simulink model "stm32f0_can_serial_bridge_binary"  (Simulink 7.3)
settings: Solver=FixedStepDiscrete  SolverMode=SingleTasking  StartTime=0.0  StopTime=10.0  RelTol=1e-3
PreLoadFcn:
  | waijung.modelPreload; % Required for working with Waijung Blockset. Do not remove.
undefined symbols (not defined in the file): LQFP48, STM32F072CB
libraries: simulink x22, stm32f0_can_lib x5, stm32f0_device_config_lib x1
(part 1 of 2)
CloseFcn:
  | waijung.modelClose; % Required for working with Waijung Blockset. Do not remove.
settings Model: Creator=Krisada  LastModifiedBy=Krisada
settings OptimizationCC: OptimizeModelRefInitCode=on  LifeSpan=1
settings HardwareCC: ProdEndianess=LittleEndian  ProdHWDeviceType=ARM Compatible->Cortex - M0  TargetEndianess=LittleEndian  TargetHWDeviceType=ARM Compatible->Cortex - M0
settings RTWCC: SystemTargetFile=stm32f0.tlc  GenerateMakefile=off  TemplateMakefile=ert_default_tmf  Description=STM32F0 Target  ProcessScript=stm32f0_make_rtw_hook
settings CodeAppCC: IgnoreCustomStorageClasses=off
settings STFCustomTargetCC: ModelReferenceCompliant=off  CombineOutputUpdateFcns=on  ERTCustomFileBanners=on  SupportContinuousTime=off  SupportNonInlinedSFcns=off  SystemTargetFile=stm32f0.tlc
settings ERTTargetCC: MultiwordLength=2048  ModelReferenceCompliant=off  ParMdlRefBuildCompliant=off  CompOptLevelCompliant=off  ERTFirstTimeCompliant=off  ModelStepFunctionPrototypeControlCompliant=off  CPPClassGenCompliant=off  ExtModeMexFile=noextcomm  InlinedParameterPlacement=NonHierarchical  ERTSrcFileBannerTemplate=stm32f0_code_template.cgt  ERTHdrFileBannerTemplate=stm32f0_code_template.cgt  ERTDataSrcFileTemplate=stm32f0_code_template.cgt  ERTDataHdrFileTemplate=stm32f0_code_template.cgt  ERTCustomFileTemplate=stm32f0_file_process.tlc

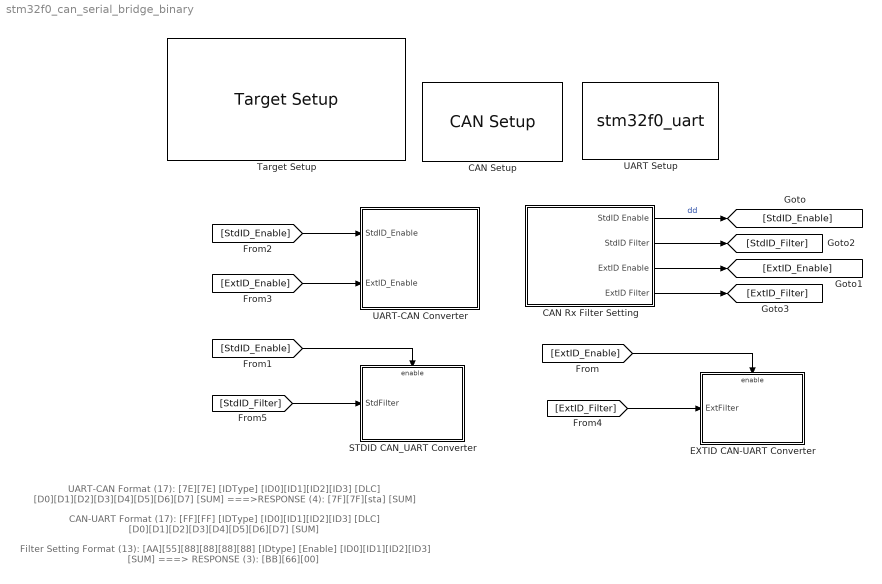
== system stm32f0_can_serial_bridge_binary ==
  note: UART-CAN Format (17): [7E][7E] [IDType] [ID0][ID1][ID2][ID3] [DLC] [D0][D1][D2][D3][D4][D5][D6][D7] [SUM] ===>RESPONSE (4): [7F][7F][sta] [SUM]
  note: CAN-UART Format (17): [FF][FF] [IDType] [ID0][ID1][ID2][ID3] [DLC] [D0][D1][D2][D3][D4][D5][D6][D7] [SUM]
  note: Filter Setting Format (13): [AA][55][88][88][88][88] [IDtype] [Enable] [ID0][ID1][ID2][ID3] [SUM] ===> RESPONSE (3): [BB][66][00]
  CAN Rx Filter Setting : Subsystem
  CAN Setup : stm32f0_can_lib/CAN Setup  conf=Setup  canmodule=1  advance=on  bitrate_select=250000  sjw=1tq  bs1=15tq  bs2=8tq  timingconf=Prescaler  brp=8  bitrate=250000  tq=1.6667e-007  autoretransmission=Enable  remaptxpin=B9  remaprxpin=B8  sampletime=-1  sampletimestr=0.001  blockid=CANSetup  inputarray=[]  inputlabelarray={}  outputarray=[]  outputlabelarray={}  compat=0  confstr="[\"250000\",\"8\",\"B\",\"9\",\"B\",\"8\",\"1tq\",\"15tq\",\"8tq\",\"DISABLE\"]"  presc=8  txportstr=B  txpinstr=9  rxportstr=B  rxpinstr=8  lastmodule=1
  EXTID CAN-UART Converter : Subsystem
  STDID CAN_UART Converter : Subsystem
  Target Setup : stm32f0_device_config_lib/Target Setup  Priority=100  compiler=GNU ARM  previous_compiler=GNU ARM  mcu=STM32F072CB (LQFP48)  mcustr=STM32F072CB  stdlib=STM32F072  clockconfig=STM32F072B-DISCO Default (HSIOSC-8MHz/HCLK-48MHz)  system_stm32f0xx_c_path=F:\trunk\targets\stm32f0_target\stm32f0\utils\STM32F0xx_AN4055\stm32f0_default\hsi8mhz_pll_hclk48mhz  showmemoryconfiguration=off  stacksize=0x400  heapsize=0x200  enableautocompiledownload=on  fullchiperase=off  programmerinterface=aMG USB Connect  editctrlstr=off  compilercontrolstr=$(patsubst %, -I%, .) -mcpu=cortex-m0 -mthumb -mabi=aapcs -Wall -O3 -mfloat-abi=soft -ffunction-sections -fdata-sections -fno-strict-aliasing -fno-builtin --short-enums  assemblercontrolstr=$(patsubst %, -I%, .) -mcpu=cortex-m0 -mtune=cortex-m0 -mthumb -Wall -O3 -Wa,-amhls=$(<:.s=.lst) -D__STACK_SIZE=$(STACK_SIZE) -D__HEAP_SIZE=$(HEAP_SIZE)  linkercontrolstr="-T$(LD_SCRIPT) -Wl,-Map=$(MAP),--cref,--no-warn-mismatch -mcpu=cortex-m0 -mthumb  -Wall -O3 -mabi=aapcs -lc -specs=nosys.specs"  runafterdownload=on  execprofile=None  profileruart=3  profilerbaud=500000  profilertxpin=Not used  profilerinitstr=0.001,48000000,48000,500000,0  manualsetsampletime=on  sampletime=0.001  blockid=TargetSetup  systickreloadvalue=48000  hseval=8000000  lastprofileruart=3  hclk=48000000  flashorigin=0x8000000  flashlength=128k  ramorigin=0x20000000  ramlength=16k  useextram=off
  UART Setup : S-Function  FunctionName=stm32f0_uart  Parameters=conf,inputporttype,inputportwidth,outputporttype,outputportwidth,asciiheader,optionstring,headerstring,terminatorstring,asciidatatypestring,sampletime,blockid  EnableBusSupport=off  mask(stm32f0_uart){conf=Setup, uartmodule=1, baudrate=115200, databits=8, parity=No, stopbit=1, remaptxpin=A9, remaprxpin=A10, flowcontrol=None, remapctspin=Not used, remaprtspin=Not used, advanceoptions=on, rxbuffersize=128, txbuffersize=128, transfer=Non-Blocking, packetmode=Binary, binheader='7E 7E', binterminator='03 03', porttype_double=1, porttype_single=1, porttype_int8=0, porttype_uint8=0, porttype_int16=0, porttype_uint16=1, porttype_int32=0, porttype_uint32=0, asciiformat='%1.2f', rx_asciiterminator=CR (0x0D - "\r"), tx_asciiterminator=CR (0x0D - "\r"), storagename=<empty>, varname=, asciiheader=, sampletime=-1, enablecustomportlabel=off, cinputportlabel=de, coutputportlabel=fff,ff,sdfsd, portpinstr=0, blockid=UARTSetup, inputporttype=[], inputportwidth=[], inputportlabel={}, outputporttype=[], outputportwidth=[], outputportlabel={}, compat=0, optionstring=["1", "1", "A", "9", "1", "A", "10", "0", "*", "*", "0", "*", "*", "1", "1", "", "", "115200", "8", "No", "1", "None", "3", "2", "128", "128", "Binary", "Non-Blocking", ""], headerstring=[], terminatorstring=[], asciidatatypestring=[], lastmodule=1}
      mask prompts: conf "Configuration"; uartmodule "UART Module"; baudrate "Baud rate (bps)"; databits "Data bits"; stopbit "Stop bit"; remaptxpin "Tx pin"; remaprxpin "Rx pin"; flowcontrol "Hardware flow control"; remapctspin "HW Flow control, CTS Pin"; remaprtspin "HW Flow control, RTS Pin"; advanceoptions "Advance options"; rxbuffersize "Rx buffer size (bytes)"; txbuffersize "Tx buffer size (bytes)"; packetmode "Packet mode"; binheader "Binary header (example: '7E 7E')"; binterminator "Binary terminator (example: '03 03')"; porttype_double "Number of data port, type DOUBLE"; porttype_single "Number of data port, type SINGLE"; porttype_int8 "Number of data port, type INT8"; porttype_uint8 "Number of data port, type UINT8"; porttype_int16 "Number of data port, type INT16"; porttype_uint16 "Number of data port, type UINT16"; porttype_int32 "Number of data port, type INT32"; porttype_uint32 "Number of data port, type UINT32"; asciiformat "Ascii format"; rx_asciiterminator "End of packet"; tx_asciiterminator "End of packet"; storagename "Buffer"; varname "Var name"; asciiheader "Ascii header (printf format)"; sampletime "Sample time (sec)"; enablecustomportlabel "Enable custom port labels (Ex. In1, In2, In3)"; cinputportlabel "Custom input port labels (Ex. In1, In2, In3)"; coutputportlabel "Custom output port labels (Ex. Out1, Out2, Out3)"; portpinstr "Port Pin String"; blockid "Block ID"; inputporttype "Input Port Type"; inputportwidth "Input Port Width"; inputportlabel "Input Port Label"; outputporttype "Output Port Type"; outputportwidth "Output Port Width"; outputportlabel "Output port label"; compat "Compatibility (Reserved for future use)"; optionstring "String(s) to be passed to TLC"; lastmodule "Last module selected"
      mask help:
      | Default configuration for aMG USB Connect board:
      |  - UART module: 1
      |  - Tx pin: A9
      |  - Rx pin: A10
      |
      | Advance options
      |  - Rx buffer size (bytes): max packet length can be received via DMA.
      |  - Tx buffer size (bytes): max packet length can be transmit via DMA.
      mask init:
      | stm32f0_uart_callback('init');
      mask Help: web(fullfile(waijungdocroot,'stm32f0_uart_setup.htm'), '-browser')
      mask StyleString: popup(Setup|Tx|Rx),popup(1|2|3|4),edit,popup(8),popup(No|Odd|Even),popup(0.5|1|1.5|2),popup(Not used|A9|B6),popup(Not used|A10|B7),popup(None|RTS|CTS|RTS/CTS),popup(Not used|A11),popup(Not used|A12),checkbox,popup(16|32|64|128|256|512),popup(16|32|64|128|256|512),popup(Blocking|Non-Blocking),popup(Ascii|Binary|String Buffer),edit,edit,edit,edit,edit,edit,edit,edit,edit,edit,edit,popup(CR (0x0D - "\r")|LF (0x0A - "\n")|CRLF (0x0D 0x0A - "\r\n")),popup(CR (0x0D - "\r")|LF (0x0A - "\n")|CRLF (0x0D 0x0A - "\r\n")|None),popup(<empty>),edit,edit,edit,checkbox,edit,edit,edit,edit,edit,edit,edit,edit,edit,edit,edit,edit,edit,edit,edit,edit
      mask CallbackString: stm32f0_uart_callback('conf');|stm32f0_uart_callback('uartmodule');|||||||stm32f0_uart_callback('flowcontrol');|||stm32f0_uart_callback('advanceoptions');|||stm32f0_uart_callback('conf');|stm32f0_uart_callback('conf');|stm32f0_uart_callback('binheader');|stm32f0_uart_callback('binterminator');|||||||||stm32f0_uart_callback('asciiformat');|||stm32f0_uart_callback('storagename');|||stm32f0_uart_callback('sampletime');|stm32f0_uart_callback('enablecustomportlabel');|stm32f0_uart_callback('conf');|stm32f0_uart_callback('conf');||stm32f0_uart_callback('blockid');||||||||||||
      mask Display: text(0.5, 0.5, 'Module: USART1_Setup\nBaud (Bps): 115200\nDMA Buffer: 128/128\nTx/Rx Pin: A9/A10','ver','middle','hor','center');
  UART-CAN Converter : Subsystem
  wires:
  CAN Rx Filter Setting/1(StdID Enable) -> [StdID_Enable]  "dd"
  CAN Rx Filter Setting/3(ExtID Enable) -> [ExtID_Enable]
  CAN Rx Filter Setting/2(StdID Filter) -> [StdID_Filter]
  CAN Rx Filter Setting/4(ExtID Filter) -> [ExtID_Filter]
  [ExtID_Enable] -> EXTID CAN-UART Converter/Enable
  [StdID_Enable] -> STDID CAN_UART Converter/Enable
  [StdID_Enable] -> UART-CAN Converter/1(StdID_Enable)
  [ExtID_Enable] -> UART-CAN Converter/2(ExtID_Enable)
  [ExtID_Filter] -> EXTID CAN-UART Converter/1(ExtFilter)
  [StdID_Filter] -> STDID CAN_UART Converter/1(StdFilter)

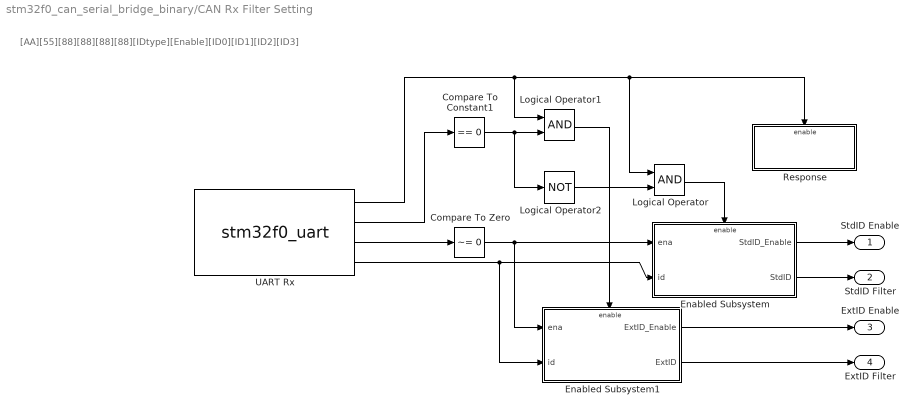
== system stm32f0_can_serial_bridge_binary/CAN Rx Filter Setting ==
  note: [AA][55][88][88][88][88][IDtype][Enable][ID0][ID1][ID2][ID3]
  Compare To Constant1 : simulink/Logic and Bit Operations/Compare To Constant  SystemSampleTime=-1  relop===  const=0  LogicOutDataTypeMode=uint8  ZeroCross=off
  Compare To Zero : simulink/Logic and Bit Operations/Compare To Zero  SystemSampleTime=-1  relop=~=  LogicOutDataTypeMode=uint8  ZeroCross=off
  Enabled Subsystem : Subsystem  TreatAsAtomicUnit=on
  Enabled Subsystem1 : Subsystem  TreatAsAtomicUnit=on
  Logical Operator : Logic  AllPortsSameDT=off  OutDataTypeMode=boolean  LogicDataType=fixdt(0, 8)  OutDataTypeStr=boolean
  Logical Operator1 : Logic  AllPortsSameDT=off  OutDataTypeMode=boolean  LogicDataType=fixdt(0, 8)  OutDataTypeStr=boolean
  Logical Operator2 : Logic  Operator=NOT  AllPortsSameDT=off  OutDataTypeMode=boolean  LogicDataType=fixdt(0, 8)  OutDataTypeStr=boolean
  Response : Subsystem  TreatAsAtomicUnit=on
  UART Rx : S-Function  FunctionName=stm32f0_uart  Parameters=conf,inputporttype,inputportwidth,outputporttype,outputportwidth,asciiheader,optionstring,headerstring,terminatorstring,asciidatatypestring,sampletime,blockid  EnableBusSupport=off  mask(stm32f0_uart){conf=Rx, uartmodule=1, baudrate=115200, databits=8, parity=No, stopbit=1, remaptxpin=A9, remaprxpin=A10, flowcontrol=None, remapctspin=Not used, remaprtspin=Not used, advanceoptions=off, rxbuffersize=64, txbuffersize=64, transfer=Non-Blocking, packetmode=Binary, binheader='AA 55 88 88 88 88', binterminator='', porttype_double=0, porttype_single=0, porttype_int8=0, porttype_uint8=2, porttype_int16=0, porttype_uint16=0, porttype_int32=0, porttype_uint32=1, asciiformat='cantx,extid=%u,dlc=%x,data=%x,%x,%x,%x,%x,%x,%x,%x', rx_asciiterminator=CRLF (0x0D 0x0A - "\r\n"), tx_asciiterminator=LF (0x0A - "\n"), storagename=<empty>, varname=, asciiheader=, sampletime=inf, enablecustomportlabel=on, cinputportlabel=de, coutputportlabel=IDtype,Enable,ID, portpinstr=0, blockid=CANRxFilterSettingUARTRx, inputporttype=[], inputportwidth=[], inputportlabel={}, outputporttype=[3 3 3 7], outputportwidth=[], outputportlabel={'READY' 'IDtype' 'Enable' 'ID'}, compat=0, optionstring=["1", "1", "A", "9", "1", "A", "10", "0", "*", "*", "0", "*", "*", "1", "1", "", "", "115200", "8", "No", "1", "None", "3", "2", "64", "64", "Binary", "Non-Blocking", ""], headerstring=["170","85","136","136","136","136"], terminatorstring=[], asciidatatypestring=[], lastmodule=1}
      mask prompts: conf "Configuration"; uartmodule "UART Module"; baudrate "Baud rate (bps)"; databits "Data bits"; stopbit "Stop bit"; remaptxpin "Tx pin"; remaprxpin "Rx pin"; flowcontrol "Hardware flow control"; remapctspin "HW Flow control, CTS Pin"; remaprtspin "HW Flow control, RTS Pin"; advanceoptions "Advance options"; rxbuffersize "Rx buffer size (bytes)"; txbuffersize "Tx buffer size (bytes)"; packetmode "Packet mode"; binheader "Binary header (example: '7E 7E')"; binterminator "Binary terminator (example: '03 03')"; porttype_double "Number of data port, type DOUBLE"; porttype_single "Number of data port, type SINGLE"; porttype_int8 "Number of data port, type INT8"; porttype_uint8 "Number of data port, type UINT8"; porttype_int16 "Number of data port, type INT16"; porttype_uint16 "Number of data port, type UINT16"; porttype_int32 "Number of data port, type INT32"; porttype_uint32 "Number of data port, type UINT32"; asciiformat "Ascii format"; rx_asciiterminator "End of packet"; tx_asciiterminator "End of packet"; storagename "Buffer"; varname "Var name"; asciiheader "Ascii header (printf format)"; sampletime "Sample time (sec)"; enablecustomportlabel "Enable custom port labels (Ex. In1, In2, In3)"; cinputportlabel "Custom input port labels (Ex. In1, In2, In3)"; coutputportlabel "Custom output port labels (Ex. Out1, Out2, Out3)"; portpinstr "Port Pin String"; blockid "Block ID"; inputporttype "Input Port Type"; inputportwidth "Input Port Width"; inputportlabel "Input Port Label"; outputporttype "Output Port Type"; outputportwidth "Output Port Width"; outputportlabel "Output port label"; compat "Compatibility (Reserved for future use)"; optionstring "String(s) to be passed to TLC"; lastmodule "Last module selected"
      mask help:
      | UART Module
      |  - Select module corresponding to "UART Setup" block.
      | Transfer
      |  - Blocking: the block wait until data receiving is ready.
      |  - Non-Blocking: if data receiving is ready, the block return non-zero to READY port otherwise return 0.
      | Packet mode:
      |  - Ascii: receiving data is ascii, Ascii format + End of packet.
      |  - Binary: receiving data is binary format, Header + Data + Terminator
      |  - String Buffer: Receiving data stored into Volatile Data Storage variable block.
      | Ascii format:
      |  - %U, %I, %D, %O, %X, %u, %i, %d, %o, %x: Uint32
      |  - %E, %G, %F, %e, %g, %f: Single
      |  - %C, %c: Int8
      mask init:
      | stm32f0_uart_callback('init');
      mask Help: web(fullfile(waijungdocroot,'stm32f0_uart_rx.htm'), '-browser')
      mask StyleString: popup(Setup|Tx|Rx),popup(1|2|3|4),edit,popup(8),popup(No|Odd|Even),popup(0.5|1|1.5|2),popup(Not used|A9|B6),popup(Not used|A10|B7),popup(None|RTS|CTS|RTS/CTS),popup(Not used|A11),popup(Not used|A12),checkbox,popup(16|32|64|128|256|512),popup(16|32|64|128|256|512),popup(Blocking|Non-Blocking),popup(Ascii|Binary|String Buffer),edit,edit,edit,edit,edit,edit,edit,edit,edit,edit,edit,popup(CR (0x0D - "\r")|LF (0x0A - "\n")|CRLF (0x0D 0x0A - "\r\n")),popup(CR (0x0D - "\r")|LF (0x0A - "\n")|CRLF (0x0D 0x0A - "\r\n")|None),popup(<empty>),edit,edit,edit,checkbox,edit,edit,edit,edit,edit,edit,edit,edit,edit,edit,edit,edit,edit,edit,edit,edit
      mask CallbackString: stm32f0_uart_callback('conf');|stm32f0_uart_callback('uartmodule');|||||||stm32f0_uart_callback('flowcontrol');|||stm32f0_uart_callback('advanceoptions');|||stm32f0_uart_callback('conf');|stm32f0_uart_callback('conf');|stm32f0_uart_callback('binheader');|stm32f0_uart_callback('binterminator');|||||||||stm32f0_uart_callback('asciiformat');|||stm32f0_uart_callback('storagename');|||stm32f0_uart_callback('sampletime');|stm32f0_uart_callback('enablecustomportlabel');|stm32f0_uart_callback('conf');|stm32f0_uart_callback('conf');||stm32f0_uart_callback('blockid');||||||||||||
      mask Display: text(0.05, 0.5, 'Module: USART1_Rx\nPacket: Binary\nTransfer: Non-Blocking\nTs (sec): 0.001','ver','middle','hor','left'); port_label('output', 1,'READY'); port_label('output', 2,'IDtype'); port_label('output', 3,'Enable'); port_label('output', 4,'ID');
  StdID Enable : Outport  OutDataType=fixdt(1, 16)  OutScaling=2^0
  StdID Filter : Outport  Port=2  OutDataType=fixdt(1, 16)  OutScaling=2^0
  ExtID Enable : Outport  Port=3  OutDataType=fixdt(1, 16)  OutScaling=2^0
  ExtID Filter : Outport  Port=4  OutDataType=fixdt(1, 16)  OutScaling=2^0
  wires:
  UART Rx/2 -> Compare To Constant1/1
  Logical Operator/1 -> Enabled Subsystem/Enable
  UART Rx/3 -> Compare To Zero/1
  UART Rx/4 -> Enabled Subsystem/2(id), Enabled Subsystem1/2(id)
  Compare To Constant1/1 -> Logical Operator1/2, Logical Operator2/1
  UART Rx/1 -> Logical Operator1/1, Logical Operator/1, Response/Enable
  Enabled Subsystem1/2(ExtID) -> ExtID Filter/1
  Enabled Subsystem1/1(ExtID_Enable) -> ExtID Enable/1
  Enabled Subsystem/2(StdID) -> StdID Filter/1
  Enabled Subsystem/1(StdID_Enable) -> StdID Enable/1
  Logical Operator2/1 -> Logical Operator/2
  Compare To Zero/1 -> Enabled Subsystem/1(ena), Enabled Subsystem1/1(ena)
  Logical Operator1/1 -> Enabled Subsystem1/Enable

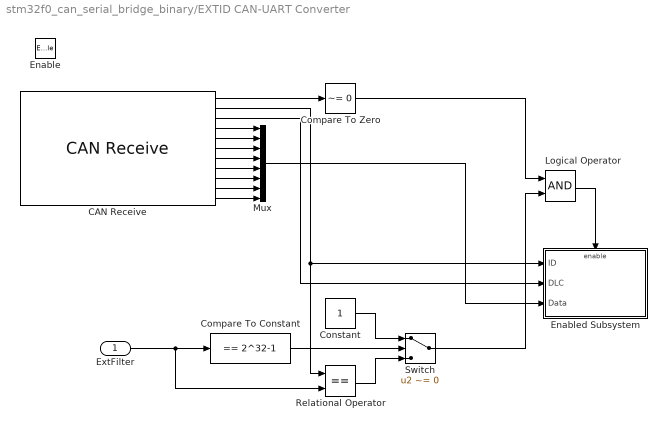
== system stm32f0_can_serial_bridge_binary/EXTID CAN-UART Converter ==
  ExtFilter : Inport  OutDataType=fixdt(1, 16)  OutScaling=2^0
  Enable : EnablePort
  CAN Receive : stm32f0_can_lib/CAN Receive  conf=Rx  canmodule=1  idtype=Extended  filtertype=Mask  id=0  idmask=0  enableisr=off  usedlc=on  datatype=single  data0type=uint8  data1type=uint8  data2type=uint8  data3type=uint8  data4type=uint8  data5type=uint8  data6type=uint8  data7type=uint8  buffersize=8  sampletime=inf  sampletimestr=0.001  blockid=EXTIDCANUARTConverterCANReceive  inputarray=[]  inputlabelarray={}  outputarray=[ 5, 7, 3, 3, 3, 3, 3, 3, 3, 3, 3]  outputlabelarray={ 'Msg Pending','ID','DLC', 'D0 (uint8)', 'D1 (uint8)', 'D2 (uint8)', 'D3 (uint8)', 'D4 (uint8)', 'D5 (uint8)', 'D6 (uint8)', 'D7 (uint8)' }  compat=0  confstr="[\"Extended\",\"Mask\",\"0\",\"0\",\"on\",\"uint8\",\"uint8\",\"uint8\",\"uint8\",\"uint8\",\"uint8\",\"uint8\",\"uint8\",\"8\",\"0\",\"4\",\"0\",\"4\"]"
  Compare To Constant : simulink/Logic and Bit Operations/Compare To Constant  SystemSampleTime=-1  relop===  const=2^32-1  LogicOutDataTypeMode=uint8  ZeroCross=off
  Compare To Zero : simulink/Logic and Bit Operations/Compare To Zero  SystemSampleTime=-1  relop=~=  LogicOutDataTypeMode=uint8  ZeroCross=off
  Constant : Constant  OutDataTypeMode=uint8  OutDataType=fixdt(1, 16)  OutScaling=2^0  OutDataTypeStr=uint8
  Enabled Subsystem : Subsystem  TreatAsAtomicUnit=on
  Logical Operator : Logic  AllPortsSameDT=off  OutDataTypeMode=boolean  LogicDataType=fixdt(0, 8)  OutDataTypeStr=boolean
  Mux : Mux  Inputs=8
  Relational Operator : RelationalOperator  Operator===  LogicOutDataTypeMode=boolean  LogicDataType=fixdt(0, 8)  OutDataTypeStr=boolean
  Switch : Switch  Criteria=u2 ~= 0  OutDataType=fixdt(1, 16)  OutScaling=2^0
  wires:
  CAN Receive/1 -> Compare To Zero/1
  CAN Receive/2 -> Enabled Subsystem/1(ID), Relational Operator/1
  CAN Receive/3 -> Enabled Subsystem/2(DLC)
  CAN Receive/4 -> Mux/1
  CAN Receive/5 -> Mux/2
  CAN Receive/6 -> Mux/3
  CAN Receive/7 -> Mux/4
  CAN Receive/8 -> Mux/5
  CAN Receive/9 -> Mux/6
  CAN Receive/10 -> Mux/7
  CAN Receive/11 -> Mux/8
  Mux/1 -> Enabled Subsystem/3(Data)
  Logical Operator/1 -> Enabled Subsystem/Enable
  Compare To Zero/1 -> Logical Operator/1
  Switch/1 -> Logical Operator/2
  ExtFilter/1 -> Compare To Constant/1, Relational Operator/2
  Compare To Constant/1 -> Switch/2
  Constant/1 -> Switch/1
  Relational Operator/1 -> Switch/3

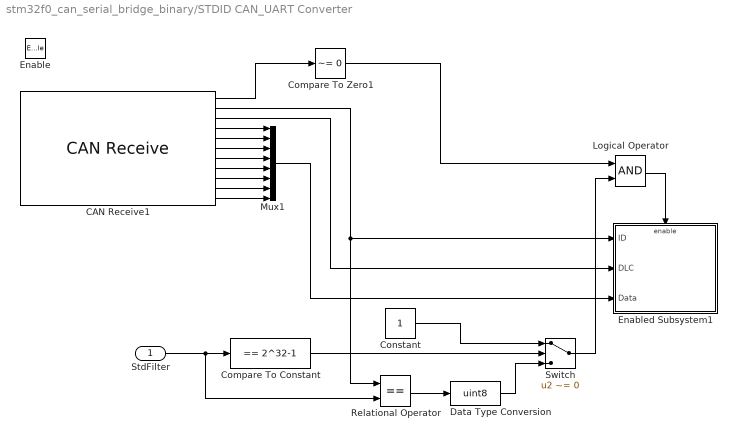
== system stm32f0_can_serial_bridge_binary/STDID CAN_UART Converter ==
  StdFilter : Inport  OutDataType=fixdt(1, 16)  OutScaling=2^0
  Enable : EnablePort
  CAN Receive1 : stm32f0_can_lib/CAN Receive  conf=Rx  canmodule=1  idtype=Standard  filtertype=Mask  id=0  idmask=0  enableisr=off  usedlc=on  datatype=single  data0type=uint8  data1type=uint8  data2type=uint8  data3type=uint8  data4type=uint8  data5type=uint8  data6type=uint8  data7type=uint8  buffersize=8  sampletime=inf  sampletimestr=0.001  blockid=STDIDCAN_UARTConverterCANReceive1  inputarray=[]  inputlabelarray={}  outputarray=[ 5, 7, 3, 3, 3, 3, 3, 3, 3, 3, 3]  outputlabelarray={ 'Msg Pending','ID','DLC', 'D0 (uint8)', 'D1 (uint8)', 'D2 (uint8)', 'D3 (uint8)', 'D4 (uint8)', 'D5 (uint8)', 'D6 (uint8)', 'D7 (uint8)' }  compat=0  confstr="[\"Standard\",\"Mask\",\"0\",\"0\",\"on\",\"uint8\",\"uint8\",\"uint8\",\"uint8\",\"uint8\",\"uint8\",\"uint8\",\"uint8\",\"8\",\"0\",\"0\",\"0\",\"4\"]"
  Compare To Constant : simulink/Logic and Bit Operations/Compare To Constant  SystemSampleTime=-1  relop===  const=2^32-1  LogicOutDataTypeMode=uint8  ZeroCross=off
  Compare To Zero1 : simulink/Logic and Bit Operations/Compare To Zero  SystemSampleTime=-1  relop=~=  LogicOutDataTypeMode=uint8  ZeroCross=off
  Constant : Constant  OutDataTypeMode=uint8  OutDataType=fixdt(1, 16)  OutScaling=2^0  OutDataTypeStr=uint8
  Data Type Conversion : DataTypeConversion  OutDataTypeMode=uint8  OutDataType=fixdt(1, 16)  OutScaling=2^0  OutDataTypeStr=uint8
  Enabled Subsystem1 : Subsystem  TreatAsAtomicUnit=on
  Logical Operator : Logic  AllPortsSameDT=off  OutDataTypeMode=boolean  LogicDataType=fixdt(0, 8)  OutDataTypeStr=boolean
  Mux1 : Mux  Inputs=8
  Relational Operator : RelationalOperator  Operator===  LogicOutDataTypeMode=boolean  LogicDataType=fixdt(0, 8)  OutDataTypeStr=boolean
  Switch : Switch  Criteria=u2 ~= 0  OutDataType=fixdt(1, 16)  OutScaling=2^0
  wires:
  CAN Receive1/1 -> Compare To Zero1/1
  CAN Receive1/4 -> Mux1/1
  CAN Receive1/5 -> Mux1/2
  CAN Receive1/6 -> Mux1/3
  CAN Receive1/7 -> Mux1/4
  CAN Receive1/8 -> Mux1/5
  CAN Receive1/9 -> Mux1/6
  CAN Receive1/10 -> Mux1/7
  CAN Receive1/11 -> Mux1/8
  CAN Receive1/2 -> Enabled Subsystem1/1(ID), Relational Operator/1
  Mux1/1 -> Enabled Subsystem1/3(Data)
  CAN Receive1/3 -> Enabled Subsystem1/2(DLC)
  Logical Operator/1 -> Enabled Subsystem1/Enable
  Compare To Zero1/1 -> Logical Operator/1
  Relational Operator/1 -> Data Type Conversion/1
  Switch/1 -> Logical Operator/2
  StdFilter/1 -> Compare To Constant/1, Relational Operator/2
  Compare To Constant/1 -> Switch/2
  Constant/1 -> Switch/1
  Data Type Conversion/1 -> Switch/3

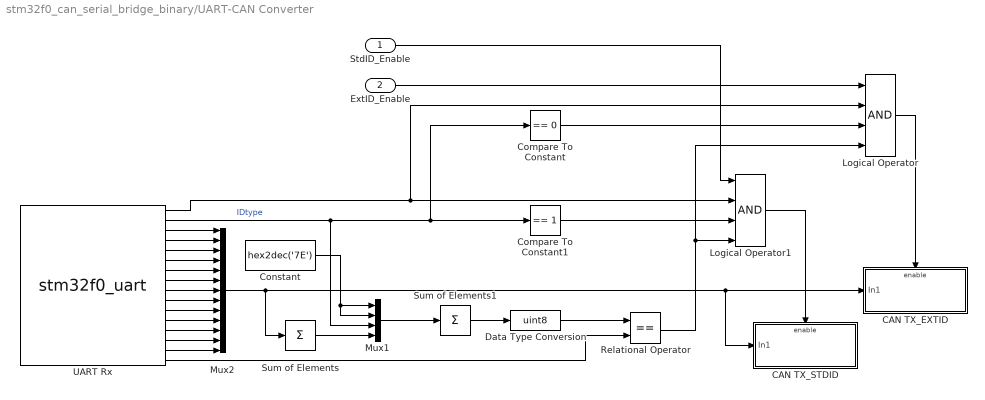
== system stm32f0_can_serial_bridge_binary/UART-CAN Converter ==
  StdID_Enable : Inport  OutDataType=fixdt(1, 16)  OutScaling=2^0
  ExtID_Enable : Inport  Port=2  OutDataType=fixdt(1, 16)  OutScaling=2^0
  CAN TX_EXTID : Subsystem  TreatAsAtomicUnit=on
  CAN TX_STDID : Subsystem  TreatAsAtomicUnit=on
  Compare To Constant : simulink/Logic and Bit Operations/Compare To Constant  SystemSampleTime=-1  relop===  const=0  LogicOutDataTypeMode=uint8  ZeroCross=off
  Compare To Constant1 : simulink/Logic and Bit Operations/Compare To Constant  SystemSampleTime=-1  relop===  const=1  LogicOutDataTypeMode=uint8  ZeroCross=off
  Constant : Constant  Value=hex2dec('7E')  OutDataTypeMode=uint8  OutDataType=fixdt(1, 16)  OutScaling=2^0  OutDataTypeStr=uint8
  Data Type Conversion : DataTypeConversion  OutDataTypeMode=uint8  OutDataType=fixdt(1, 16)  OutScaling=2^0  OutDataTypeStr=uint8
  Logical Operator : Logic  Inputs=4  AllPortsSameDT=off  OutDataTypeMode=boolean  LogicDataType=fixdt(0, 8)  OutDataTypeStr=boolean
  Logical Operator1 : Logic  Inputs=4  AllPortsSameDT=off  OutDataTypeMode=boolean  LogicDataType=fixdt(0, 8)  OutDataTypeStr=boolean
  Mux1 : Mux
  Mux2 : Mux  Inputs=13
  Relational Operator : RelationalOperator  Operator===  LogicOutDataTypeMode=boolean  LogicDataType=fixdt(0, 8)  OutDataTypeStr=boolean
  Sum of Elements : Sum  Inputs=+  OutDataType=fixdt(1, 16)  OutScaling=2^-10
  Sum of Elements1 : Sum  Inputs=+  OutDataType=fixdt(1, 16)  OutScaling=2^-10
  UART Rx : S-Function  FunctionName=stm32f0_uart  Parameters=conf,inputporttype,inputportwidth,outputporttype,outputportwidth,asciiheader,optionstring,headerstring,terminatorstring,asciidatatypestring,sampletime,blockid  EnableBusSupport=off  mask(stm32f0_uart){conf=Rx, uartmodule=1, baudrate=115200, databits=8, parity=No, stopbit=1, remaptxpin=A9, remaprxpin=A10, flowcontrol=None, remapctspin=Not used, remaprtspin=Not used, advanceoptions=off, rxbuffersize=64, txbuffersize=64, transfer=Non-Blocking, packetmode=Binary, binheader='7E 7E', binterminator='', porttype_double=0, porttype_single=0, porttype_int8=0, porttype_uint8=15, porttype_int16=0, porttype_uint16=0, porttype_int32=0, porttype_uint32=0, asciiformat='cantx,extid=%u,dlc=%x,data=%x,%x,%x,%x,%x,%x,%x,%x', rx_asciiterminator=CRLF (0x0D 0x0A - "\r\n"), tx_asciiterminator=LF (0x0A - "\n"), storagename=<empty>, varname=, asciiheader=, sampletime=inf, enablecustomportlabel=off, cinputportlabel=de, coutputportlabel=fff,ff,sdfsd, portpinstr=0, blockid=UARTCANConverterUARTRx, inputporttype=[], inputportwidth=[], inputportlabel={}, outputporttype=[3 3 3 3 3 3 3 3 3 3 3 3 3 3 3 3], outputportwidth=[], outputportlabel={'READY' 'uint8' 'uint8' 'uint8' 'uint8' 'uint8' 'uint8' 'uint8' 'uint8' 'uint8' 'uint8' 'uint8' 'uint8' 'uint8' 'uint8' 'uint8'}, compat=0, optionstring=["1", "1", "A", "9", "1", "A", "10", "0", "*", "*", "0", "*", "*", "1", "1", "", "", "115200", "8", "No", "1", "None", "3", "2", "64", "64", "Binary", "Non-Blocking", ""], headerstring=["126","126"], terminatorstring=[], asciidatatypestring=[], lastmodule=1}
      mask prompts: conf "Configuration"; uartmodule "UART Module"; baudrate "Baud rate (bps)"; databits "Data bits"; stopbit "Stop bit"; remaptxpin "Tx pin"; remaprxpin "Rx pin"; flowcontrol "Hardware flow control"; remapctspin "HW Flow control, CTS Pin"; remaprtspin "HW Flow control, RTS Pin"; advanceoptions "Advance options"; rxbuffersize "Rx buffer size (bytes)"; txbuffersize "Tx buffer size (bytes)"; packetmode "Packet mode"; binheader "Binary header (example: '7E 7E')"; binterminator "Binary terminator (example: '03 03')"; porttype_double "Number of data port, type DOUBLE"; porttype_single "Number of data port, type SINGLE"; porttype_int8 "Number of data port, type INT8"; porttype_uint8 "Number of data port, type UINT8"; porttype_int16 "Number of data port, type INT16"; porttype_uint16 "Number of data port, type UINT16"; porttype_int32 "Number of data port, type INT32"; porttype_uint32 "Number of data port, type UINT32"; asciiformat "Ascii format"; rx_asciiterminator "End of packet"; tx_asciiterminator "End of packet"; storagename "Buffer"; varname "Var name"; asciiheader "Ascii header (printf format)"; sampletime "Sample time (sec)"; enablecustomportlabel "Enable custom port labels (Ex. In1, In2, In3)"; cinputportlabel "Custom input port labels (Ex. In1, In2, In3)"; coutputportlabel "Custom output port labels (Ex. Out1, Out2, Out3)"; portpinstr "Port Pin String"; blockid "Block ID"; inputporttype "Input Port Type"; inputportwidth "Input Port Width"; inputportlabel "Input Port Label"; outputporttype "Output Port Type"; outputportwidth "Output Port Width"; outputportlabel "Output port label"; compat "Compatibility (Reserved for future use)"; optionstring "String(s) to be passed to TLC"; lastmodule "Last module selected"
      mask help:
      | UART Module
      |  - Select module corresponding to "UART Setup" block.
      | Transfer
      |  - Blocking: the block wait until data receiving is ready.
      |  - Non-Blocking: if data receiving is ready, the block return non-zero to READY port otherwise return 0.
      | Packet mode:
      |  - Ascii: receiving data is ascii, Ascii format + End of packet.
      |  - Binary: receiving data is binary format, Header + Data + Terminator
      |  - String Buffer: Receiving data stored into Volatile Data Storage variable block.
      | Ascii format:
      |  - %U, %I, %D, %O, %X, %u, %i, %d, %o, %x: Uint32
      |  - %E, %G, %F, %e, %g, %f: Single
      |  - %C, %c: Int8
      mask init:
      | stm32f0_uart_callback('init');
      mask Help: web(fullfile(waijungdocroot,'stm32f0_uart_rx.htm'), '-browser')
      mask StyleString: popup(Setup|Tx|Rx),popup(1|2|3|4),edit,popup(8),popup(No|Odd|Even),popup(0.5|1|1.5|2),popup(Not used|A9|B6),popup(Not used|A10|B7),popup(None|RTS|CTS|RTS/CTS),popup(Not used|A11),popup(Not used|A12),checkbox,popup(16|32|64|128|256|512),popup(16|32|64|128|256|512),popup(Blocking|Non-Blocking),popup(Ascii|Binary|String Buffer),edit,edit,edit,edit,edit,edit,edit,edit,edit,edit,edit,popup(CR (0x0D - "\r")|LF (0x0A - "\n")|CRLF (0x0D 0x0A - "\r\n")),popup(CR (0x0D - "\r")|LF (0x0A - "\n")|CRLF (0x0D 0x0A - "\r\n")|None),popup(<empty>),edit,edit,edit,checkbox,edit,edit,edit,edit,edit,edit,edit,edit,edit,edit,edit,edit,edit,edit,edit,edit
      mask CallbackString: stm32f0_uart_callback('conf');|stm32f0_uart_callback('uartmodule');|||||||stm32f0_uart_callback('flowcontrol');|||stm32f0_uart_callback('advanceoptions');|||stm32f0_uart_callback('conf');|stm32f0_uart_callback('conf');|stm32f0_uart_callback('binheader');|stm32f0_uart_callback('binterminator');|||||||||stm32f0_uart_callback('asciiformat');|||stm32f0_uart_callback('storagename');|||stm32f0_uart_callback('sampletime');|stm32f0_uart_callback('enablecustomportlabel');|stm32f0_uart_callback('conf');|stm32f0_uart_callback('conf');||stm32f0_uart_callback('blockid');||||||||||||
      mask Display: text(0.05, 0.5, 'Module: USART1_Rx\nPacket: Binary\nTransfer: Non-Blocking\nTs (sec): 0.001','ver','middle','hor','left'); port_label('output', 1,'READY'); port_label('output', 2,'uint8'); port_label('output', 3,'uint8'); port_label('output', 4,'uint8'); port_label('output', 5,'uint8'); port_label('output', 6,'uint8'); port_label('output', 7,'uint8'); port_label('output', 8,'uint8'); port_label('output', 9,'uint8'); port_label('output', 10,'uint8'); port_label('output', 11,'uint8'); port_label('output', 12,'uint8'); port_label('output', 13,'uint8'); port_label('output', 14,'uint8'); port_label('output', 15,'uint8'); port_label('output', 16,'uint8');
  wires:
  UART Rx/1 -> Logical Operator/2, Logical Operator1/2
  Mux2/1 -> CAN TX_EXTID/1(In1), CAN TX_STDID/1(In1), Sum of Elements/1
  Logical Operator/1 -> CAN TX_EXTID/Enable
  UART Rx/2 -> Compare To Constant/1, Compare To Constant1/1, Mux1/3  "IDtype"
  Logical Operator1/1 -> CAN TX_STDID/Enable
  Compare To Constant/1 -> Logical Operator/3
  ExtID_Enable/1 -> Logical Operator/1
  Compare To Constant1/1 -> Logical Operator1/3
  StdID_Enable/1 -> Logical Operator1/1
  UART Rx/3 -> Mux2/1
  UART Rx/4 -> Mux2/2
  UART Rx/5 -> Mux2/3
  UART Rx/6 -> Mux2/4
  UART Rx/7 -> Mux2/5
  UART Rx/8 -> Mux2/6
  UART Rx/9 -> Mux2/7
  UART Rx/10 -> Mux2/8
  UART Rx/11 -> Mux2/9
  UART Rx/12 -> Mux2/10
  UART Rx/13 -> Mux2/11
  UART Rx/14 -> Mux2/12
  UART Rx/15 -> Mux2/13
  Sum of Elements/1 -> Mux1/4
  Constant/1 -> Mux1/1, Mux1/2
  Mux1/1 -> Sum of Elements1/1
  Sum of Elements1/1 -> Data Type Conversion/1
  Data Type Conversion/1 -> Relational Operator/1
  UART Rx/16 -> Relational Operator/2
  Relational Operator/1 -> Logical Operator1/4, Logical Operator/4

== system stm32f0_can_serial_bridge_binary/CAN Rx Filter Setting/Enabled Subsystem ==
  ena : Inport  OutDataType=fixdt(1, 16)  OutScaling=2^0
  id : Inport  Port=2  OutDataType=fixdt(1, 16)  OutScaling=2^0
  Enable : EnablePort
  StdID_Enable : Outport  OutDataType=fixdt(1, 16)  OutScaling=2^0  InitialOutput=0
  StdID : Outport  Port=2  OutDataType=fixdt(1, 16)  OutScaling=2^0  InitialOutput=2^32-1
  wires:
  ena/1 -> StdID_Enable/1
  id/1 -> StdID/1

== system stm32f0_can_serial_bridge_binary/CAN Rx Filter Setting/Enabled Subsystem1 ==
  ena : Inport  OutDataType=fixdt(1, 16)  OutScaling=2^0
  id : Inport  Port=2  OutDataType=fixdt(1, 16)  OutScaling=2^0
  Enable : EnablePort
  ExtID_Enable : Outport  OutDataType=fixdt(1, 16)  OutScaling=2^0  InitialOutput=0
  ExtID : Outport  Port=2  OutDataType=fixdt(1, 16)  OutScaling=2^0  InitialOutput=2^32-1
  wires:
  id/1 -> ExtID/1
  ena/1 -> ExtID_Enable/1

== system stm32f0_can_serial_bridge_binary/CAN Rx Filter Setting/Response ==
  note: [BB][66][00]
  Enable : EnablePort
  UART Tx : S-Function  FunctionName=stm32f0_uart  Parameters=conf,inputporttype,inputportwidth,outputporttype,outputportwidth,asciiheader,optionstring,headerstring,terminatorstring,asciidatatypestring,sampletime,blockid  EnableBusSupport=off  mask(stm32f0_uart){conf=Tx, uartmodule=1, baudrate=115200, databits=8, parity=No, stopbit=1, remaptxpin=A9, remaprxpin=A10, flowcontrol=None, remapctspin=Not used, remaprtspin=Not used, advanceoptions=off, rxbuffersize=64, txbuffersize=64, transfer=Blocking, packetmode=Binary, binheader='BB 66 00', binterminator='', porttype_double=0, porttype_single=0, porttype_int8=0, porttype_uint8=0, porttype_int16=0, porttype_uint16=0, porttype_int32=0, porttype_uint32=0, asciiformat='%u: CODE: %u', rx_asciiterminator=CR (0x0D - "\r"), tx_asciiterminator=CRLF (0x0D 0x0A - "\r\n"), storagename=<empty>, varname=, asciiheader=, sampletime=inf, enablecustomportlabel=off, cinputportlabel=de, coutputportlabel=fff,ff,sdfsd, portpinstr=0, blockid=CANRxFilterSettingResponseUARTTx, inputporttype=[], inputportwidth=[], inputportlabel={}, outputporttype=[], outputportwidth=[], outputportlabel={}, compat=0, optionstring=["1", "1", "A", "9", "1", "A", "10", "0", "*", "*", "0", "*", "*", "1", "1", "", "", "115200", "8", "No", "1", "None", "3", "2", "64", "64", "Binary", "Blocking", ""], headerstring=["187","102","0"], terminatorstring=[], asciidatatypestring=[], lastmodule=1}
      mask prompts: conf "Configuration"; uartmodule "UART Module"; baudrate "Baud rate (bps)"; databits "Data bits"; stopbit "Stop bit"; remaptxpin "Tx pin"; remaprxpin "Rx pin"; flowcontrol "Hardware flow control"; remapctspin "HW Flow control, CTS Pin"; remaprtspin "HW Flow control, RTS Pin"; advanceoptions "Advance options"; rxbuffersize "Rx buffer size (bytes)"; txbuffersize "Tx buffer size (bytes)"; packetmode "Packet mode"; binheader "Binary header (example: '7E 7E')"; binterminator "Binary terminator (example: '03 03')"; porttype_double "Number of data port, type DOUBLE"; porttype_single "Number of data port, type SINGLE"; porttype_int8 "Number of data port, type INT8"; porttype_uint8 "Number of data port, type UINT8"; porttype_int16 "Number of data port, type INT16"; porttype_uint16 "Number of data port, type UINT16"; porttype_int32 "Number of data port, type INT32"; porttype_uint32 "Number of data port, type UINT32"; asciiformat "Ascii format"; rx_asciiterminator "End of packet"; tx_asciiterminator "End of packet"; storagename "Buffer"; varname "Var name"; asciiheader "Ascii header (printf format)"; sampletime "Sample time (sec)"; enablecustomportlabel "Enable custom port labels (Ex. In1, In2, In3)"; cinputportlabel "Custom input port labels (Ex. In1, In2, In3)"; coutputportlabel "Custom output port labels (Ex. Out1, Out2, Out3)"; portpinstr "Port Pin String"; blockid "Block ID"; inputporttype "Input Port Type"; inputportwidth "Input Port Width"; inputportlabel "Input Port Label"; outputporttype "Output Port Type"; outputportwidth "Output Port Width"; outputportlabel "Output port label"; compat "Compatibility (Reserved for future use)"; optionstring "String(s) to be passed to TLC"; lastmodule "Last module selected"
      mask help:
      | UART Module
      |  - Select module corresponding to "UART Setup" block.
      | Transfer
      |  - Blocking: after write DMA buffer, the block wait until buffer empty.
      |  - Non-Blocking: the block will not wait for buffer empty.
      | Packet mode:
      |  - Ascii: sending data is ascii, Ascii format + End of packet.
      |  - Binary: sending data is binary format, Header + Data + Terminator
      |  - String Buffer: Volatile Data Storage variable name as sending data.
      | Ascii format:
      |  - %U, %I, %D, %O, %X, %u, %i, %d, %o, %x: Uint32
      |  - %E, %G, %F, %e, %g, %f: Single
      |  - %C, %c: Int8
      |  - %S, %s: (char *), this port is output of Volatile Data Storage Read block, which data type is string.
      mask init:
      | stm32f0_uart_callback('init');
      mask Help: web(fullfile(waijungdocroot,'stm32f0_uart_tx.htm'), '-browser')
      mask StyleString: popup(Setup|Tx|Rx),popup(1|2|3|4),edit,popup(8),popup(No|Odd|Even),popup(0.5|1|1.5|2),popup(Not used|A9|B6),popup(Not used|A10|B7),popup(None|RTS|CTS|RTS/CTS),popup(Not used|A11),popup(Not used|A12),checkbox,popup(16|32|64|128|256|512),popup(16|32|64|128|256|512),popup(Blocking|Non-Blocking),popup(Ascii|Binary|String Buffer),edit,edit,edit,edit,edit,edit,edit,edit,edit,edit,edit,popup(CR (0x0D - "\r")|LF (0x0A - "\n")|CRLF (0x0D 0x0A - "\r\n")),popup(CR (0x0D - "\r")|LF (0x0A - "\n")|CRLF (0x0D 0x0A - "\r\n")|None),popup(<empty>),edit,edit,edit,checkbox,edit,edit,edit,edit,edit,edit,edit,edit,edit,edit,edit,edit,edit,edit,edit,edit
      mask CallbackString: stm32f0_uart_callback('conf');|stm32f0_uart_callback('uartmodule');|||||||stm32f0_uart_callback('flowcontrol');|||stm32f0_uart_callback('advanceoptions');|||stm32f0_uart_callback('conf');|stm32f0_uart_callback('conf');|stm32f0_uart_callback('binheader');|stm32f0_uart_callback('binterminator');|||||||||stm32f0_uart_callback('asciiformat');|||stm32f0_uart_callback('storagename');|||stm32f0_uart_callback('sampletime');|stm32f0_uart_callback('enablecustomportlabel');|stm32f0_uart_callback('conf');|stm32f0_uart_callback('conf');||stm32f0_uart_callback('blockid');||||||||||||
      mask Display: text(0.95, 0.5, 'Module: USART1_Tx\nPacket: Binary\nTransfer: Blocking\nTs (sec): 0.001','ver','middle','hor','right');

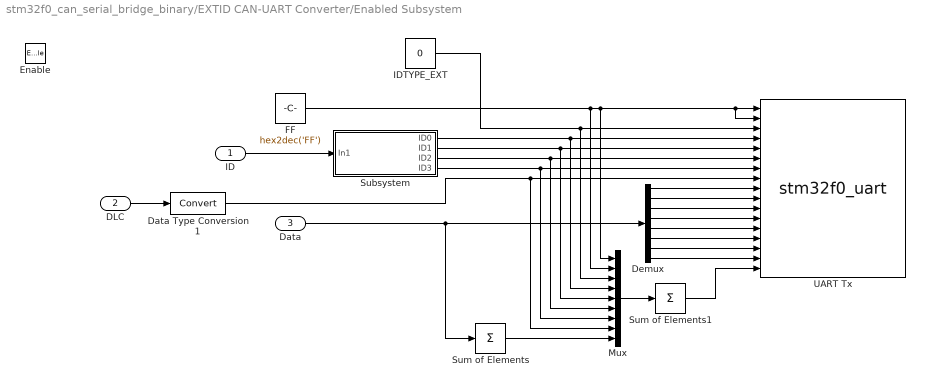
== system stm32f0_can_serial_bridge_binary/EXTID CAN-UART Converter/Enabled Subsystem ==
  ID : Inport  OutDataType=fixdt(1, 16)  OutScaling=2^0
  DLC : Inport  Port=2  OutDataType=fixdt(1, 16)  OutScaling=2^0
  Data : Inport  Port=3  OutDataType=fixdt(1, 16)  OutScaling=2^0
  Enable : EnablePort
  Data Type Conversion1 : DataTypeConversion  OutDataType=fixdt(1, 16)  OutScaling=2^0
  Demux : Demux  Outputs=8
  FF : Constant  Value=hex2dec('FF')  OutDataTypeMode=uint8  OutDataType=fixdt(1, 16)  OutScaling=2^0  OutDataTypeStr=uint8
  IDTYPE_EXT : Constant  Value=0  OutDataTypeMode=uint8  OutDataType=fixdt(1, 16)  OutScaling=2^0  OutDataTypeStr=uint8
  Mux : Mux  Inputs=9
  Subsystem : Subsystem
  Sum of Elements : Sum  Inputs=+  OutDataType=fixdt(1, 16)  OutScaling=2^-10
  Sum of Elements1 : Sum  Inputs=+  OutDataType=fixdt(1, 16)  OutScaling=2^-10
  UART Tx : S-Function  FunctionName=stm32f0_uart  Parameters=conf,inputporttype,inputportwidth,outputporttype,outputportwidth,asciiheader,optionstring,headerstring,terminatorstring,asciidatatypestring,sampletime,blockid  EnableBusSupport=off  mask(stm32f0_uart){conf=Tx, uartmodule=1, baudrate=115200, databits=8, parity=No, stopbit=1, remaptxpin=A9, remaprxpin=A10, flowcontrol=None, remapctspin=Not used, remaprtspin=Not used, advanceoptions=off, rxbuffersize=64, txbuffersize=64, transfer=Blocking, packetmode=Binary, binheader='', binterminator='', porttype_double=0, porttype_single=0, porttype_int8=0, porttype_uint8=17, porttype_int16=0, porttype_uint16=0, porttype_int32=0, porttype_uint32=0, asciiformat='%u,canrx,extid=%u,dlc=%u,data=%x,%x,%x,%x,%x,%x,%x,%x', rx_asciiterminator=CR (0x0D - "\r"), tx_asciiterminator=CRLF (0x0D 0x0A - "\r\n"), storagename=<empty>, varname=, asciiheader=, sampletime=inf, enablecustomportlabel=off, cinputportlabel=de, coutputportlabel=fff,ff,sdfsd, portpinstr=0, blockid=EXTIDCANUARTConverterEnabledSubsystemUARTTx, inputporttype=[3 3 3 3 3 3 3 3 3 3 3 3 3 3 3 3 3], inputportwidth=[], inputportlabel={'uint8' 'uint8' 'uint8' 'uint8' 'uint8' 'uint8' 'uint8' 'uint8' 'uint8' 'uint8' 'uint8' 'uint8' 'uint8' 'uint8' 'uint8' 'uint8' 'uint8'}, outputporttype=[], outputportwidth=[], outputportlabel={}, compat=0, optionstring=["1", "1", "A", "9", "1", "A", "10", "0", "*", "*", "0", "*", "*", "1", "1", "", "", "115200", "8", "No", "1", "None", "3", "2", "64", "64", "Binary", "Blocking", ""], headerstring=[], terminatorstring=[], asciidatatypestring=[], lastmodule=1}
      mask prompts: conf "Configuration"; uartmodule "UART Module"; baudrate "Baud rate (bps)"; databits "Data bits"; stopbit "Stop bit"; remaptxpin "Tx pin"; remaprxpin "Rx pin"; flowcontrol "Hardware flow control"; remapctspin "HW Flow control, CTS Pin"; remaprtspin "HW Flow control, RTS Pin"; advanceoptions "Advance options"; rxbuffersize "Rx buffer size (bytes)"; txbuffersize "Tx buffer size (bytes)"; packetmode "Packet mode"; binheader "Binary header (example: '7E 7E')"; binterminator "Binary terminator (example: '03 03')"; porttype_double "Number of data port, type DOUBLE"; porttype_single "Number of data port, type SINGLE"; porttype_int8 "Number of data port, type INT8"; porttype_uint8 "Number of data port, type UINT8"; porttype_int16 "Number of data port, type INT16"; porttype_uint16 "Number of data port, type UINT16"; porttype_int32 "Number of data port, type INT32"; porttype_uint32 "Number of data port, type UINT32"; asciiformat "Ascii format"; rx_asciiterminator "End of packet"; tx_asciiterminator "End of packet"; storagename "Buffer"; varname "Var name"; asciiheader "Ascii header (printf format)"; sampletime "Sample time (sec)"; enablecustomportlabel "Enable custom port labels (Ex. In1, In2, In3)"; cinputportlabel "Custom input port labels (Ex. In1, In2, In3)"; coutputportlabel "Custom output port labels (Ex. Out1, Out2, Out3)"; portpinstr "Port Pin String"; blockid "Block ID"; inputporttype "Input Port Type"; inputportwidth "Input Port Width"; inputportlabel "Input Port Label"; outputporttype "Output Port Type"; outputportwidth "Output Port Width"; outputportlabel "Output port label"; compat "Compatibility (Reserved for future use)"; optionstring "String(s) to be passed to TLC"; lastmodule "Last module selected"
      mask help:
      | UART Module
      |  - Select module corresponding to "UART Setup" block.
      | Transfer
      |  - Blocking: after write DMA buffer, the block wait until buffer empty.
      |  - Non-Blocking: the block will not wait for buffer empty.
      | Packet mode:
      |  - Ascii: sending data is ascii, Ascii format + End of packet.
      |  - Binary: sending data is binary format, Header + Data + Terminator
      |  - String Buffer: Volatile Data Storage variable name as sending data.
      | Ascii format:
      |  - %U, %I, %D, %O, %X, %u, %i, %d, %o, %x: Uint32
      |  - %E, %G, %F, %e, %g, %f: Single
      |  - %C, %c: Int8
      |  - %S, %s: (char *), this port is output of Volatile Data Storage Read block, which data type is string.
      mask init:
      | stm32f0_uart_callback('init');
      mask Help: web(fullfile(waijungdocroot,'stm32f0_uart_tx.htm'), '-browser')
      mask StyleString: popup(Setup|Tx|Rx),popup(1|2|3|4),edit,popup(8),popup(No|Odd|Even),popup(0.5|1|1.5|2),popup(Not used|A9|B6),popup(Not used|A10|B7),popup(None|RTS|CTS|RTS/CTS),popup(Not used|A11),popup(Not used|A12),checkbox,popup(16|32|64|128|256|512),popup(16|32|64|128|256|512),popup(Blocking|Non-Blocking),popup(Ascii|Binary|String Buffer),edit,edit,edit,edit,edit,edit,edit,edit,edit,edit,edit,popup(CR (0x0D - "\r")|LF (0x0A - "\n")|CRLF (0x0D 0x0A - "\r\n")),popup(CR (0x0D - "\r")|LF (0x0A - "\n")|CRLF (0x0D 0x0A - "\r\n")|None),popup(<empty>),edit,edit,edit,checkbox,edit,edit,edit,edit,edit,edit,edit,edit,edit,edit,edit,edit,edit,edit,edit,edit
      mask CallbackString: stm32f0_uart_callback('conf');|stm32f0_uart_callback('uartmodule');|||||||stm32f0_uart_callback('flowcontrol');|||stm32f0_uart_callback('advanceoptions');|||stm32f0_uart_callback('conf');|stm32f0_uart_callback('conf');|stm32f0_uart_callback('binheader');|stm32f0_uart_callback('binterminator');|||||||||stm32f0_uart_callback('asciiformat');|||stm32f0_uart_callback('storagename');|||stm32f0_uart_callback('sampletime');|stm32f0_uart_callback('enablecustomportlabel');|stm32f0_uart_callback('conf');|stm32f0_uart_callback('conf');||stm32f0_uart_callback('blockid');||||||||||||
      mask Display: text(0.95, 0.5, 'Module: USART1_Tx\nPacket: Binary\nTransfer: Blocking\nTs (sec): 0.001','ver','middle','hor','right'); port_label('input', 1,'uint8'); port_label('input', 2,'uint8'); port_label('input', 3,'uint8'); port_label('input', 4,'uint8'); port_label('input', 5,'uint8'); port_label('input', 6,'uint8'); port_label('input', 7,'uint8'); port_label('input', 8,'uint8'); port_label('input', 9,'uint8'); port_label('input', 10,'uint8'); port_label('input', 11,'uint8'); port_label('input', 12,'uint8'); port_label('input', 13,'uint8'); port_label('input', 14,'uint8'); port_label('input', 15,'uint8'); port_label('input', 16,'uint8'); port_label('input', 17,'uint8');
  wires:
  DLC/1 -> Data Type Conversion1/1
  FF/1 -> UART Tx/1, UART Tx/2, Mux/1, Mux/2
  IDTYPE_EXT/1 -> UART Tx/3, Mux/3
  Subsystem/1(ID0) -> UART Tx/4, Mux/4
  Subsystem/2(ID1) -> UART Tx/5, Mux/5
  Subsystem/3(ID2) -> UART Tx/6, Mux/6
  Subsystem/4(ID3) -> UART Tx/7, Mux/7
  ID/1 -> Subsystem/1(In1)
  Data Type Conversion1/1 -> UART Tx/8, Mux/8
  Demux/1 -> UART Tx/9
  Demux/2 -> UART Tx/10
  Demux/3 -> UART Tx/11
  Demux/4 -> UART Tx/12
  Demux/5 -> UART Tx/13
  Demux/6 -> UART Tx/14
  Demux/7 -> UART Tx/15
  Demux/8 -> UART Tx/16
  Data/1 -> Demux/1, Sum of Elements/1
  Sum of Elements/1 -> Mux/9
  Mux/1 -> Sum of Elements1/1
  Sum of Elements1/1 -> UART Tx/17
